simulink model "SF045A_HwAgSysArbn"  (R2013b)
settings: Solver=FixedStepDiscrete  SolverMode=SingleTasking  StartTime=0.0  StopTime=1  FixedStep=.002  RelTol=1e-3
values from neighbouring files (symbols this model uses):
  ARCHGLBPRM_2MILLISEC_SEC_F32 = DataDict.Constant    [SF045A_HwAgSysArbn_DataDict.m]
  ARCHGLBPRM_FLOATZEROTHD_ULS_F32 = DataDict.Constant    [SF045A_HwAgSysArbn_DataDict.m]
  ARCHGLBPRM_PIOVER180_ULS_F32 = DataDict.Constant    [SF045A_HwAgSysArbn_DataDict.m]
  CNVSECTOCNT_ULS_U32 = DataDict.Constant    [SF045A_HwAgSysArbn_DataDict.m]
  CNVTOMILLISEC_MILLISECPERCNT_F32 = DataDict.Constant    [SF045A_HwAgSysArbn_DataDict.m]
  FltInj_f32 = DataDict.Client    [SF045A_HwAgSysArbn_DataDict.m]
  FLTINJ_HWAGSYSARBN_HWAG = DataDict.Constant    [SF045A_HwAgSysArbn_DataDict.m]
  FLTINJ_HWAGSYSARBN_SERLCOMHWAG = DataDict.Constant    [SF045A_HwAgSysArbn_DataDict.m]
  HwAgCorrlnFlt = DataDict.NTC    [SF045A_HwAgSysArbn_DataDict.m]
  HwAgSnsrlsThdExcdd = DataDict.NTC    [SF045A_HwAgSysArbn_DataDict.m]
  HwAgSysArbnHwAgConf1Snsr = DataDict.Calibration    [SF045A_HwAgSysArbn_DataDict.m]
  HwAgSysArbnHwAgConf2Snsr = DataDict.Calibration    [SF045A_HwAgSysArbn_DataDict.m]
  HwAgSysArbnHwAgConfNoSnsr = DataDict.Calibration    [SF045A_HwAgSysArbn_DataDict.m]
  HwAgSysArbnHwAgCorrdCorrlnThd = DataDict.Calibration    [SF045A_HwAgSysArbn_DataDict.m]
  HwAgSysArbnHwAgCorrlnFailDebStep = DataDict.Calibration    [SF045A_HwAgSysArbn_DataDict.m]
  HwAgSysArbnHwAgCorrlnPassDebStep = DataDict.Calibration    [SF045A_HwAgSysArbn_DataDict.m]
  HwAgSysArbnHwAgCorrlnRng = DataDict.Calibration    [SF045A_HwAgSysArbn_DataDict.m]
  HwAgSysArbnHwAgSlewRate = DataDict.Calibration    [SF045A_HwAgSysArbn_DataDict.m]
  HwAgSysArbnHwAgSnsrlsCorrlnThd = DataDict.Calibration    [SF045A_HwAgSysArbn_DataDict.m]
  HwAgSysArbnHwAgSnsrlsKineThd = DataDict.Calibration    [SF045A_HwAgSysArbn_DataDict.m]
  HwAgSysArbnHwAgToMotAgCorrlnElpdTiLim = DataDict.Calibration    [SF045A_HwAgSysArbn_DataDict.m]
  HwAgSysArbnSerlComHwAgCorrdConf = DataDict.Calibration    [SF045A_HwAgSysArbn_DataDict.m]
  HwAgSysArbnSerlComHwAgSnsrlsConf = DataDict.Calibration    [SF045A_HwAgSysArbn_DataDict.m]
  HwAgSysArbnSlewRateTmr = DataDict.Calibration    [SF045A_HwAgSysArbn_DataDict.m]
  HWAGTHD_ULS_FLOAT32 = DataDict.Constant    [SF045A_HwAgSysArbn_DataDict.m]
  INVLDSRC_CNT_S08 = DataDict.Constant    [SF045A_HwAgSysArbn_DataDict.m]
  LRGSLEW_HWDEGPERSEC_F32 = DataDict.Constant    [SF045A_HwAgSysArbn_DataDict.m]
  NODEBSTEP_CNT_U16 = DataDict.Constant    [SF045A_HwAgSysArbn_DataDict.m]
  SLEWINPROGS_CNT_LGC = DataDict.Constant    [SF045A_HwAgSysArbn_DataDict.m]
  SLEWNOTINPROGS_CNT_LGC = DataDict.Constant    [SF045A_HwAgSysArbn_DataDict.m]
  SNSRDATASRCSELD_CNT_S08 = DataDict.Constant    [SF045A_HwAgSysArbn_DataDict.m]
  SNSRLSDATASRCSELD_CNT_S08 = DataDict.Constant    [SF045A_HwAgSysArbn_DataDict.m]
  SysGlbPrmSysKineRat = DataDict.ImprtdCal    [SF045A_HwAgSysArbn_DataDict.m]
  SysGlbPrmTorsBarStfn = DataDict.ImprtdCal    [SF045A_HwAgSysArbn_DataDict.m]
  ZEROTMR_MILLISEC_F32 = DataDict.Constant    [SF045A_HwAgSysArbn_DataDict.m]
undefined symbols (not defined in the file or in its folder): NtcSts1
libraries: NxtrLim x11, simulink x6, NxtrAbslt x6, Fil x3, autosarlib x2
(part 1 of 6)
settings Model: PauseTimes=0.48  CovFilter=UTP_SF045A_HwAgSysArbn_cov_flt_list  CovHTMLOptions=-sRT=1 -aTS=1 -bRG=1 -bTC=1 -hTR=0 -nFC=0 -scm=1 -bcm=1 -xEv=0  Creator=TZ5743  LastModifiedBy=NZ2883
settings SolverCC: AutoInsertRateTranBlk=on  InsertRTBMode=Always
settings DataIOCC: LimitDataPoints=off  SaveFormat=Structure  ReturnWorkspaceOutputs=on
settings OptimizationCC: BlockReduction=off  InlineParams=on  ZeroExternalMemoryAtStartup=off  ZeroInternalMemoryAtStartup=off  OptimizeModelRefInitCode=on  LifeSpan=1
settings DebuggingCC: SignalInfNanChecking=error  SignalRangeChecking=warning  UnderspecifiedInitializationDetection=Simplified  SolverPrmCheckMsg=error  InheritedTsInSrcMsg=error  DiscreteInheritContinuousMsg=error  SingleTaskRateTransMsg=error  TasksWithSamePriorityMsg=error  SigSpecEnsureSampleTimeMsg=error  CheckMatrixSingularityMsg=error  ParameterUnderflowMsg=error  ParameterPrecisionLossMsg=error  ParameterTunabilityLossMsg=error  FixptConstUnderflowMsg=warning  FixptConstOverflowMsg=warning  VectorMatrixConversionMsg=error  SignalLabelMismatchMsg=error  UnconnectedInputMsg=error  UnconnectedOutputMsg=error  UnconnectedLineMsg=error  SFcnCompatibilityMsg=error  UniqueDataStoreMsg=warning  BusObjectLabelMismatch=error  RootOutportRequireBusObject=error  AssertControl=DisableAll  ModelReferenceIOMsg=error  ModelReferenceVersionMismatchMessage=warning  ModelReferenceIOMismatchMessage=error  ModelReferenceCSMismatchMessage=warning  ModelReferenceDataLoggingMessage=error  StateNameClashWarn=warning  StrictBusMsg=ErrorOnBusTreatedAsVector  NonBusSignalsTreatedAsBus=error  SFUnexpectedBacktrackingDiag=error  SFInvalidInputDataAccessInChartInitDiag=error  SFNoUnconditionalDefaultTransitionDiag=error  SFTransitionOutsideNaturalParentDiag=error  SFUnconditionalTransitionShadowingDiag=error  SFUndirectedBroadcastEventsDiag=error
settings ModelReferenceCC: ModelReferenceNumInstancesAllowed=Single
settings RTWCC: SystemTargetFile=autosar.tlc  GenCodeOnly=on  TemplateMakefile=ert_default_tmf  Description=AUTOSAR  GenerateReport=on  ProcessScript=autosar_make_rtw_hook  LaunchReport=on
settings CodeAppCC: GenerateComments=off  IgnoreCustomStorageClasses=off  CustomSymbolStrType=$N$R$M  CustomSymbolStrBlkIO=$N$M  SimulinkBlockComments=off
settings STFCustomTargetCC: ParMdlRefBuildCompliant=on  CompOptLevelCompliant=on  IncludeMdlTerminateFcn=off  CombineOutputUpdateFcns=on  SuppressErrorStatus=on  ERTFirstTimeCompliant=on  ERTCustomFileBanners=on  SupportNonFinite=off  SupportComplex=off  SupportContinuousTime=off  SupportNonInlinedSFcns=off  MATLABClassNameForMDSCustomization=Simulink.SoftwareTarget.ERTCustomization  AutosarCompliant=on  GRTInterface=off  SystemTargetFile=autosar.tlc
settings ERTTargetCC: CodeReplacementLibrary=ANSI_C  ConcurrentExecutionCompliant=off  IncludeMdlTerminateFcn=off  SuppressErrorStatus=on  SupportNonFinite=off  SupportComplex=off  ModelStepFunctionPrototypeControlCompliant=off  CPPClassGenCompliant=off  AutosarCompliant=on  InlinedParameterPlacement=NonHierarchical  ERTCustomFileTemplate=example_file_process.tlc  EnableUserReplacementTypes=on

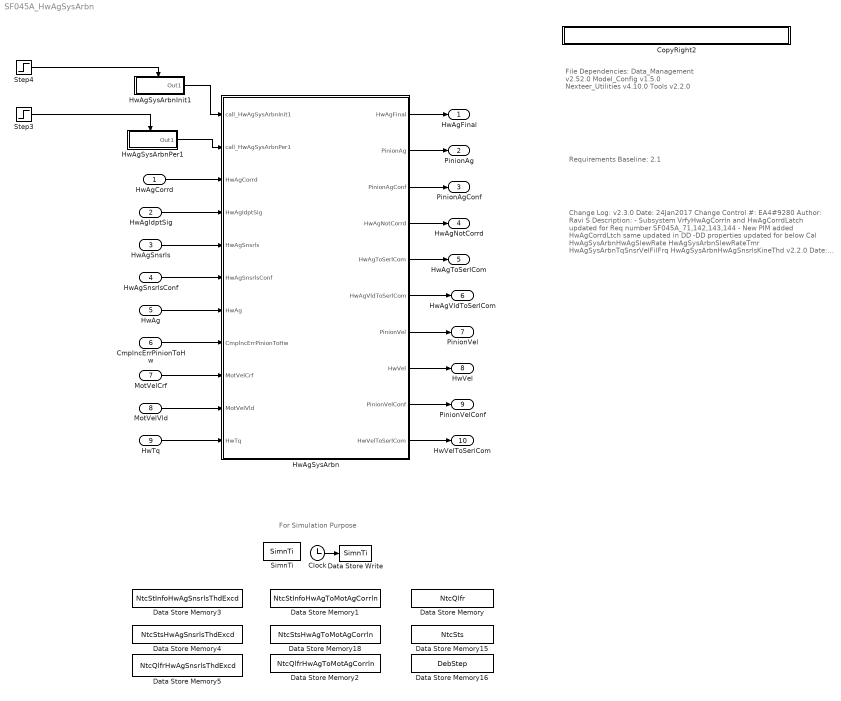
== system SF045A_HwAgSysArbn ==
  note: For Simulation Purpose
  note: File Dependencies:
      |
      | Data_Management v2.52.0
      | Model_Config v1.5.0
      | Nexteer_Utilities v4.10.0
      | Tools v2.2.0
  note: Requirements Baseline: 2.1
  note: Change Log:
      |
      | v2.3.0
      | Date: 24Jan2017
      | Change Control #: EA4#9280
      | Author: Ravi S
      | Description:
      | - Subsystem VrfyHwAgCorrln and HwAgCorrdLatch updated for
      |   Req number SF045A_71,142,143,144
      | - New PIM added HwAgCorrdLtch same updated in DD
      | -DD properties updated for below Cal
      |     HwAgSysArbnHwAgSlewRate
      |     HwAgSysArbnSlewRateTmr
      |     HwAgSysArbnTqSnsrVelFilFrq
      |     HwAgSysArbnHwAgSnsrlsKineThd
      |
      |
      | v2.2.0
      | Date: 29Nov2016
      | Change Control #: EA4#8582
      | Author: Ravi S
      | Description:
      | - MotorVelocityVld subsystem updated to compute
      |   HwVel = MotVelCrf / kinematic ratio.
      |
      |
      |
      |
      | v2.1.0
      | Date: 22-Nov-16
      | Change Control#: EA4#8179
      | Author:Ravi S
      | Description :
      | - Subsystem HwAgVelSeriCom and CalcPinionVel added .
      | - Subsystem HwAgSeriCom earlier was present in HwAgSrcSeln,
      |   which now repositioned  and added logig for Handwheel Velocity
      |   Serial Com.
      | - Requirements links added to all sub-systems
      |
      |
      | v2.0.0
      | Date: 15-Jun-16
      | Change Control#: EA4#5839
      | Author: Sudeep Shankar
      | Description :
      | - Generic design is now simplified considering only Pinion
      | coordinates to arbitrate the HwAg signals instead of flexibility to
      | choose between Handwheel, Pinion or MotorAg coordinates.
      | This resulted in removing the cals used to apply compilance error
      | compensation and priority selection.
      | - Kinematic Integrity diagonstic added
      | - HwAg to MotAg Correlation diagonstic added
      | - Logic added to arbitrate HwAg signal going to EOT when HwAg
      | sensor signals not available.
      |
      | v1.1.0
      | Date: 12-Sep-2015
      | Change Control #: EA4#860
      | Author:  Sudeep Shankar
      | Description:
      | - Minor modification in source change logic
      |  detection to avoid ambiguity in state variable
      |  read and write priorities
      | - Setting Initial condition of while loop to 'true'
      | instead of comparing greater than 1.
      | - Removed signal conversion blocks wherever
      | not required.
      | - Set while loop iteration to '-1' instead of restricting
      | it to '5' as condition check is in place to restrict
      | while iteration equal to number of signals present.
      |
      | v1.0.0
      | Date: 28-Aug-2015
      | Change Control #: EA4#860
      | Author:  Sudeep Shankar
      | Description:
      | - EA4 Initial Release
  HwAgCorrd : Inport  RequirementInfo={} %GIDa_cc9a7bcf_75f9_45c8_a24f_b8479fae80cf
  HwAgIdptSig : Inport  RequirementInfo={} %GIDa_9a7b919a_3c4b_44c1_bb96_545a47b8b3d3  Port=2
  HwAgSnsrls : Inport  RequirementInfo={} %GIDa_eede448f_64dd_4146_b16f_6fc16ca31f60  Port=3
  HwAgSnsrlsConf : Inport  RequirementInfo={} %GIDa_f6d9b3ed_9576_46cf_8319_2d07116884b2  Port=4
  HwAg : Inport  RequirementInfo={} %GIDa_3ab8439e_d791_45cf_9b38_dc1d6a5d96c4  Port=5
  CmplncErrPinionToHw : Inport  RequirementInfo={} %GIDa_8afc3a2b_29a0_4b25_ac8f_049b17fb3d6a  Port=6
  MotVelCrf : Inport  Port=7
  MotVelVld : Inport  Port=8
  HwTq : Inport  Port=9
  Clock : Clock
  CopyRight2 : Subsystem  Description=|  mask(Copyright Information){none=on}
      | Copyright info block.                                               
      |                                                                     
      | Place copyright information at the top of every subsystem in design.
      mask prompts: none "No parameters"
      mask help: Place copyright information at the top of every subsystem in design.
      mask Display:
      | NxtrConf = 'Nexteer Confidential';
      | 
      | sys = bdroot; %handle for the current model ("system")
      | first = get_param(sys,'Created');
      | first = first(end-3:end);  %year is last four digits
      | 
      | last = get_param(sys,'LastModifiedDate');
      | if isempty(last)
      |     last = datestr(now,'yyyy');
      | else
      |     last = last(end-3:end);
      | end
      | 
      | if strcmp(first,last)
      |     fprintf('%s -- Copyright %s Nexteer',NxtrConf,first)
      | else
      |     fprintf('%s -- %s%s- %s Nexteer',NxtrConf,char(169),first,last)
      | end
  Data Store Memory : DataStoreMemory  DataStoreName=NtcQlfr  InitialValue=SigQlfr1.SIGQLFR_NORES  OutDataTypeStr=Enum: SigQlfr1
  Data Store Memory1 : DataStoreMemory  DataStoreName=NtcStInfoHwAgToMotAgCorrln  OutDataTypeStr=uint8
  Data Store Memory15 : DataStoreMemory  DataStoreName=NtcSts  InitialValue=NtcSts1.NTCSTS_PREPASSD  OutDataTypeStr=Enum: NtcSts1
  Data Store Memory16 : DataStoreMemory  DataStoreName=DebStep
  Data Store Memory18 : DataStoreMemory  DataStoreName=NtcStsHwAgToMotAgCorrln  InitialValue=NtcSts1.NTCSTS_PASSD  OutDataTypeStr=Enum: NtcSts1
  Data Store Memory2 : DataStoreMemory  DataStoreName=NtcQlfrHwAgToMotAgCorrln  InitialValue=SigQlfr1.SIGQLFR_NORES  OutDataTypeStr=Enum: SigQlfr1
  Data Store Memory3 : DataStoreMemory  DataStoreName=NtcStInfoHwAgSnsrlsThdExcd  OutDataTypeStr=uint8
  Data Store Memory4 : DataStoreMemory  DataStoreName=NtcStsHwAgSnsrlsThdExcd  InitialValue=NtcSts1.NTCSTS_PASSD  OutDataTypeStr=Enum: NtcSts1
  Data Store Memory5 : DataStoreMemory  DataStoreName=NtcQlfrHwAgSnsrlsThdExcd  InitialValue=SigQlfr1.SIGQLFR_NORES  OutDataTypeStr=Enum: SigQlfr1
  Data Store Write : DataStoreWrite  DataStoreName=SimnTi
  HwAgSysArbn : Subsystem  RequirementInfo="{'linktype_rmi_doors' '00012ce0 (/E-STEER Core/SubSystem Specifications/Application Functions - EA4/SF045A Handwheel Angle System Arbitration)' '#SF045A_108' 'true' 'REQ:  SF045A_108' '' } %GIDa_b3e0ed6f_fb94_4fa4_96b1_04061689a89e"
  HwAgSysArbnInit1 : Subsystem  RequirementInfo="{'linktype_rmi_doors' '00012ce0 (/E-STEER Core/SubSystem Specifications/Application Functions - EA4/SF045A Handwheel Angle System Arbitration)' '#SF045A_108' 'true' 'REQ:  SF045A_108' '' ; 'linktype_rmi_doors' '00012ce0 (/E-STEER Core/SubSystem Specifications/Application Functions - EA4/SF045A Handwheel Angle System Arbitration)' '#SF045A_34' 'true' 'REQ:  SF045A_34' '' } %GIDa_057ddbd1_6821_4128_a5e6_a444f48d7204"  TreatAsAtomicUnit=on
  HwAgSysArbnPer1 : Subsystem  RequirementInfo="{'linktype_rmi_doors' '00012ce0 (/E-STEER Core/SubSystem Specifications/Application Functions - EA4/SF045A Handwheel Angle System Arbitration)' '#SF045A_108' 'true' 'REQ:  SF045A_108' '' ; 'linktype_rmi_doors' '00012ce0 (/E-STEER Core/SubSystem Specifications/Application Functions - EA4/SF045A Handwheel Angle System Arbitration)' '#SF045A_34' 'true' 'REQ:  SF045A_34' '' } %GIDa_e117302a_b889_4d12_a49a_80c3f747018f"  TreatAsAtomicUnit=on
  SimnTi : DataStoreMemory  DataStoreName=SimnTi
  Step3 : Step  Time=0  SampleTime=0.002
  Step4 : Step  Time=0  Before=1  After=0  SampleTime=0.002
  HwAgFinal : Outport
  PinionAg : Outport  Port=2
  PinionAgConf : Outport  Port=3
  HwAgNotCorrd : Outport  Port=4
  HwAgToSerlCom : Outport  Port=5
  HwAgVldToSerlCom : Outport  Port=6
  PinionVel : Outport  Port=7
  HwVel : Outport  Port=8
  PinionVelConf : Outport  Port=9
  HwVelToSeriCom : Outport  Port=10
  wires:
  HwAgSysArbn/2(PinionAg) -> PinionAg/1
  HwAgSysArbn/3(PinionAgConf) -> PinionAgConf/1
  HwAgSysArbn/4(HwAgNotCorrd) -> HwAgNotCorrd/1
  HwAgSysArbn/1(HwAgFinal) -> HwAgFinal/1
  HwAgSysArbn/6(HwAgVldToSerlCom) -> HwAgVldToSerlCom/1
  Clock/1 -> Data Store Write/1
  HwAgSysArbn/5(HwAgToSerlCom) -> HwAgToSerlCom/1
  HwAgSysArbnInit1/1(Out1) -> HwAgSysArbn/1(call_HwAgSysArbnInit1)
  HwAgSysArbnPer1/1(Out1) -> HwAgSysArbn/2(call_HwAgSysArbnPer1)
  HwAgSnsrls/1 -> HwAgSysArbn/5(HwAgSnsrls)
  HwAgCorrd/1 -> HwAgSysArbn/3(HwAgCorrd)
  HwAgSnsrlsConf/1 -> HwAgSysArbn/6(HwAgSnsrlsConf)
  HwAgIdptSig/1 -> HwAgSysArbn/4(HwAgIdptSig)
  CmplncErrPinionToHw/1 -> HwAgSysArbn/8(CmplncErrPinionToHw)
  HwAg/1 -> HwAgSysArbn/7(HwAg)
  Step3/1 -> HwAgSysArbnPer1/Enable
  MotVelCrf/1 -> HwAgSysArbn/9(MotVelCrf)
  MotVelVld/1 -> HwAgSysArbn/10(MotVelVld)
  HwTq/1 -> HwAgSysArbn/11(HwTq)
  HwAgSysArbn/7(PinionVel) -> PinionVel/1
  HwAgSysArbn/8(HwVel) -> HwVel/1
  HwAgSysArbn/9(PinionVelConf) -> PinionVelConf/1
  HwAgSysArbn/10(HwVelToSerlCom) -> HwVelToSeriCom/1
  Step4/1 -> HwAgSysArbnInit1/Enable

== system SF045A_HwAgSysArbn/CopyRight2 ==

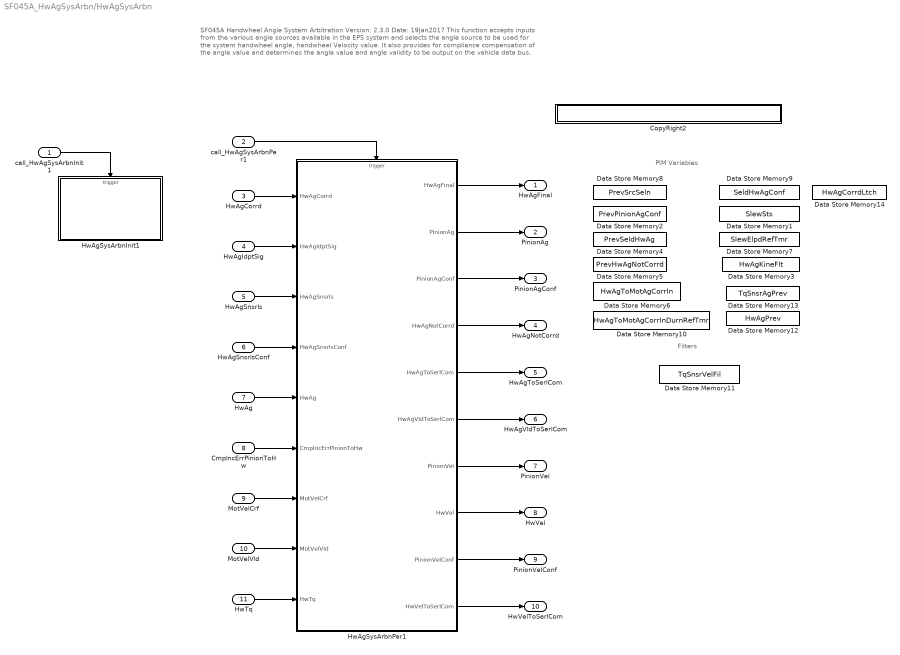
== system SF045A_HwAgSysArbn/HwAgSysArbn ==
  note: PIM Variables
  note: SF045A  Handwheel Angle System Arbitration       Version: 2.3.0                                                        Date: 19Jan2017
      |
      | This function accepts inputs from the various angle sources available in the EPS system and selects the angle
      | source to be used for the system handwheel angle, handwheel Velocity value.
      | It also provides for compliance compensation of the angle value and determines the angle value and angle validity to be output on the vehicle data bus.
  note: Filters
  call_HwAgSysArbnInit1 : Inport
  call_HwAgSysArbnPer1 : Inport  Port=2
  HwAgCorrd : Inport  RequirementInfo="{'linktype_rmi_doors' '00012ce0 (/E-STEER Core/SubSystem Specifications/Application Functions - EA4/SF045A Handwheel Angle System Arbitration)' '#SF045A_9' 'true' 'REQ:  SF045A_9' '' } %GIDa_0c48395d_f55e_4aa8_967c_ddfcd5dc0f09"  Port=3
  HwAgIdptSig : Inport  RequirementInfo="{'linktype_rmi_doors' '00012ce0 (/E-STEER Core/SubSystem Specifications/Application Functions - EA4/SF045A Handwheel Angle System Arbitration)' '#SF045A_47' 'true' 'REQ:  SF045A_47' '' } %GIDa_050c3700_87b8_4e6a_a603_fe10bf5bb98d"  Port=4
  HwAgSnsrls : Inport  RequirementInfo="{'linktype_rmi_doors' '00012ce0 (/E-STEER Core/SubSystem Specifications/Application Functions - EA4/SF045A Handwheel Angle System Arbitration)' '#SF045A_46' 'true' 'REQ:  SF045A_46' '' } %GIDa_2af70a6d_5cf9_42e5_985f_0de67760f974"  Port=5
  HwAgSnsrlsConf : Inport  RequirementInfo="{'linktype_rmi_doors' '00012ce0 (/E-STEER Core/SubSystem Specifications/Application Functions - EA4/SF045A Handwheel Angle System Arbitration)' '#SF045A_48' 'true' 'REQ:  SF045A_48' '' } %GIDa_205f4441_a425_4e75_91eb_166c28519f31"  Port=6
  HwAg : Inport  RequirementInfo="{'linktype_rmi_doors' '00012ce0 (/E-STEER Core/SubSystem Specifications/Application Functions - EA4/SF045A Handwheel Angle System Arbitration)' '#SF045A_49' 'true' 'REQ:  SF045A_49' '' } %GIDa_bd860903_e40a_4856_a107_6e65debfd627"  Port=7
  CmplncErrPinionToHw : Inport  RequirementInfo="{'linktype_rmi_doors' '00012ce0 (/E-STEER Core/SubSystem Specifications/Application Functions - EA4/SF045A Handwheel Angle System Arbitration)' '#SF045A_50' 'true' 'REQ:  SF045A_50' '' } %GIDa_fd50d5ef_7c8c_43a4_8956_a275e6267051"  Port=8
  MotVelCrf : Inport  RequirementInfo="{'linktype_rmi_doors' '00012ce0 (/E-STEER Core/SubSystem Specifications/Application Functions - EA4/SF045A Handwheel Angle System Arbitration)' '#SF045A_127' 'true' 'REQ:  SF045A_127' '' } %GIDa_90030ca0_2589_4eab_adf5_a0272c142c23"  Port=9
  MotVelVld : Inport  RequirementInfo="{'linktype_rmi_doors' '00012ce0 (/E-STEER Core/SubSystem Specifications/Application Functions - EA4/SF045A Handwheel Angle System Arbitration)' '#SF045A_128' 'true' 'REQ:  SF045A_128' '' } %GIDa_c2b99d6a_26e3_4ced_a354_7c878afdb5f5"  Port=10
  HwTq : Inport  RequirementInfo="{'linktype_rmi_doors' '00012ce0 (/E-STEER Core/SubSystem Specifications/Application Functions - EA4/SF045A Handwheel Angle System Arbitration)' '#SF045A_130' 'true' 'REQ:  SF045A_130' '' } %GIDa_722f0d6d_b063_4bab_a5a3_bad3ad3ad2ff"  Port=11
  CopyRight2 : Subsystem  Description=|  mask(Copyright Information){none=on}
      | Copyright info block.                                               
      |                                                                     
      | Place copyright information at the top of every subsystem in design.
      mask prompts: none "No parameters"
      mask help: Place copyright information at the top of every subsystem in design.
      mask Display:
      | NxtrConf = 'Nexteer Confidential';
      | 
      | sys = bdroot; %handle for the current model ("system")
      | first = get_param(sys,'Created');
      | first = first(end-3:end);  %year is last four digits
      | 
      | last = get_param(sys,'LastModifiedDate');
      | if isempty(last)
      |     last = datestr(now,'yyyy');
      | else
      |     last = last(end-3:end);
      | end
      | 
      | if strcmp(first,last)
      |     fprintf('%s -- Copyright %s Nexteer',NxtrConf,first)
      | else
      |     fprintf('%s -- %s%s- %s Nexteer',NxtrConf,char(169),first,last)
      | end
  Data Store Memory1 : DataStoreMemory  DataStoreName=SlewSts  StateMustResolveToSignalObject=on
  Data Store Memory10 : DataStoreMemory  DataStoreName=HwAgToMotAgCorrlnDurnRefTmr  StateMustResolveToSignalObject=on
  Data Store Memory11 : DataStoreMemory  DataStoreName=TqSnsrVelFil  InitialValue=[]  OutDataTypeStr=Bus: FilLpRec1  StateMustResolveToSignalObject=on
  Data Store Memory12 : DataStoreMemory  DataStoreName=HwAgPrev  StateMustResolveToSignalObject=on
  Data Store Memory13 : DataStoreMemory  DataStoreName=TqSnsrAgPrev  StateMustResolveToSignalObject=on
  Data Store Memory14 : DataStoreMemory  DataStoreName=HwAgCorrdLtch  StateMustResolveToSignalObject=on
  Data Store Memory2 : DataStoreMemory  DataStoreName=PrevPinionAgConf  StateMustResolveToSignalObject=on
  Data Store Memory3 : DataStoreMemory  DataStoreName=HwAgKineFlt  StateMustResolveToSignalObject=on
  Data Store Memory4 : DataStoreMemory  DataStoreName=PrevSeldHwAg  StateMustResolveToSignalObject=on
  Data Store Memory5 : DataStoreMemory  DataStoreName=PrevHwAgNotCorrd  StateMustResolveToSignalObject=on
  Data Store Memory6 : DataStoreMemory  DataStoreName=HwAgToMotAgCorrln  StateMustResolveToSignalObject=on
  Data Store Memory7 : DataStoreMemory  DataStoreName=SlewElpdRefTmr  StateMustResolveToSignalObject=on
  Data Store Memory8 : DataStoreMemory  DataStoreName=PrevSrcSeln  StateMustResolveToSignalObject=on
  Data Store Memory9 : DataStoreMemory  DataStoreName=SeldHwAgConf  StateMustResolveToSignalObject=on
  HwAgSysArbnInit1 : Subsystem  RequirementInfo="{'linktype_rmi_doors' '00012ce0 (/E-STEER Core/SubSystem Specifications/Application Functions - EA4/SF045A Handwheel Angle System Arbitration)' '#SF045A_34' 'true' 'REQ:  SF045A_34' '' ; 'linktype_rmi_doors' '00012ce0 (/E-STEER Core/SubSystem Specifications/Application Functions - EA4/SF045A Handwheel Angle System Arbitration)' '#SF045A_123' 'true' 'REQ:  SF045A_123' '' } %GIDa_ffe1340e_7dd3_453f_8ec7_9bdff50c1f90"  TreatAsAtomicUnit=on
  HwAgSysArbnPer1 : Subsystem  RequirementInfo="{'linktype_rmi_doors' '00012ce0 (/E-STEER Core/SubSystem Specifications/Application Functions - EA4/SF045A Handwheel Angle System Arbitration)' '#SF045A_67' 'true' 'REQ:  SF045A_67' '' } %GIDa_40c16d0c_868c_4be8_ac7a_d7644aab2a82"
  HwAgFinal : Outport  RequirementInfo="{'linktype_rmi_doors' '00012ce0 (/E-STEER Core/SubSystem Specifications/Application Functions - EA4/SF045A Handwheel Angle System Arbitration)' '#SF045A_11' 'true' 'REQ:  SF045A_11' '' } %GIDa_011fe0ec_bcc0_4a9e_bfa8_b93370ffdc5f"
  PinionAg : Outport  RequirementInfo="{'linktype_rmi_doors' '00012ce0 (/E-STEER Core/SubSystem Specifications/Application Functions - EA4/SF045A Handwheel Angle System Arbitration)' '#SF045A_51' 'true' 'REQ:  SF045A_51' '' } %GIDa_f176d339_cae7_40f0_af7d_2598900e3a6e"  Port=2
  PinionAgConf : Outport  RequirementInfo="{'linktype_rmi_doors' '00012ce0 (/E-STEER Core/SubSystem Specifications/Application Functions - EA4/SF045A Handwheel Angle System Arbitration)' '#SF045A_52' 'true' 'REQ:  SF045A_52' '' } %GIDa_ba6f2b72_e674_40ee_820e_69cfc9bdaacd"  Port=3
  HwAgNotCorrd : Outport  RequirementInfo="{'linktype_rmi_doors' '00012ce0 (/E-STEER Core/SubSystem Specifications/Application Functions - EA4/SF045A Handwheel Angle System Arbitration)' '#SF045A_55' 'true' 'REQ:  SF045A_55' '' } %GIDa_667dfd31_56c6_4848_b6a8_5a3d7a5632fb"  Port=4
  HwAgToSerlCom : Outport  RequirementInfo="{'linktype_rmi_doors' '00012ce0 (/E-STEER Core/SubSystem Specifications/Application Functions - EA4/SF045A Handwheel Angle System Arbitration)' '#SF045A_56' 'true' 'REQ:  SF045A_56' '' } %GIDa_8096249c_a6e2_4a31_b51a_c06af36d6bde"  Port=5
  HwAgVldToSerlCom : Outport  RequirementInfo="{'linktype_rmi_doors' '00012ce0 (/E-STEER Core/SubSystem Specifications/Application Functions - EA4/SF045A Handwheel Angle System Arbitration)' '#SF045A_57' 'true' 'REQ:  SF045A_57' '' } %GIDa_30b9e9dd_ad37_434a_8538_15d621b4541c"  Port=6
  PinionVel : Outport  RequirementInfo="{'linktype_rmi_doors' '00012ce0 (/E-STEER Core/SubSystem Specifications/Application Functions - EA4/SF045A Handwheel Angle System Arbitration)' '#SF045A_132' 'true' 'REQ:  SF045A_132' '' } %GIDa_825df61a_9b42_4745_9a19_f867d9578a4d"  Port=7
  HwVel : Outport  RequirementInfo="{'linktype_rmi_doors' '00012ce0 (/E-STEER Core/SubSystem Specifications/Application Functions - EA4/SF045A Handwheel Angle System Arbitration)' '#SF045A_134' 'true' 'REQ:  SF045A_134' '' } %GIDa_df719774_fce7_4f7c_868b_fd6ca13ffd9c"  Port=8
  PinionVelConf : Outport  RequirementInfo="{'linktype_rmi_doors' '00012ce0 (/E-STEER Core/SubSystem Specifications/Application Functions - EA4/SF045A Handwheel Angle System Arbitration)' '#SF045A_133' 'true' 'REQ:  SF045A_133' '' } %GIDa_5297214b_1fb7_41a8_8266_2143d92809ac"  Port=9
  HwVelToSerlCom : Outport  RequirementInfo="{'linktype_rmi_doors' '00012ce0 (/E-STEER Core/SubSystem Specifications/Application Functions - EA4/SF045A Handwheel Angle System Arbitration)' '#SF045A_135' 'true' 'REQ:  SF045A_135' '' } %GIDa_0c50da69_21aa_4d0e_a4ce_f9ea2be8a725"  Port=10
  wires:
  call_HwAgSysArbnPer1/1 -> HwAgSysArbnPer1/Trigger
  call_HwAgSysArbnInit1/1 -> HwAgSysArbnInit1/Trigger
  HwAgSysArbnPer1/4(HwAgNotCorrd) -> HwAgNotCorrd/1
  HwAgSysArbnPer1/2(PinionAg) -> PinionAg/1
  HwAgSysArbnPer1/6(HwAgVldToSerlCom) -> HwAgVldToSerlCom/1
  HwAgSysArbnPer1/5(HwAgToSerlCom) -> HwAgToSerlCom/1
  HwAgSysArbnPer1/3(PinionAgConf) -> PinionAgConf/1
  HwAgSnsrls/1 -> HwAgSysArbnPer1/3(HwAgSnsrls)
  HwAgCorrd/1 -> HwAgSysArbnPer1/1(HwAgCorrd)
  HwAgSnsrlsConf/1 -> HwAgSysArbnPer1/4(HwAgSnsrlsConf)
  HwAgIdptSig/1 -> HwAgSysArbnPer1/2(HwAgIdptSig)
  CmplncErrPinionToHw/1 -> HwAgSysArbnPer1/6(CmplncErrPinionToHw)
  HwAg/1 -> HwAgSysArbnPer1/5(HwAg)
  HwAgSysArbnPer1/1(HwAgFinal) -> HwAgFinal/1
  MotVelCrf/1 -> HwAgSysArbnPer1/7(MotVelCrf)
  MotVelVld/1 -> HwAgSysArbnPer1/8(MotVelVld)
  HwTq/1 -> HwAgSysArbnPer1/9(HwTq)
  HwAgSysArbnPer1/7(PinionVel) -> PinionVel/1
  HwAgSysArbnPer1/8(HwVel) -> HwVel/1
  HwAgSysArbnPer1/9(PinionVelConf) -> PinionVelConf/1
  HwAgSysArbnPer1/10(HwVelToSerlCom) -> HwVelToSerlCom/1

== system SF045A_HwAgSysArbn/HwAgSysArbnInit1 ==
  Enable : EnablePort
  CopyRight2 : Subsystem  Description=|  mask(Copyright Information){none=on}
      | Copyright info block.                                               
      |                                                                     
      | Place copyright information at the top of every subsystem in design.
      mask prompts: none "No parameters"
      mask help: Place copyright information at the top of every subsystem in design.
      mask Display:
      | NxtrConf = 'Nexteer Confidential';
      | 
      | sys = bdroot; %handle for the current model ("system")
      | first = get_param(sys,'Created');
      | first = first(end-3:end);  %year is last four digits
      | 
      | last = get_param(sys,'LastModifiedDate');
      | if isempty(last)
      |     last = datestr(now,'yyyy');
      | else
      |     last = last(end-3:end);
      | end
      | 
      | if strcmp(first,last)
      |     fprintf('%s -- Copyright %s Nexteer',NxtrConf,first)
      | else
      |     fprintf('%s -- %s%s- %s Nexteer',NxtrConf,char(169),first,last)
      | end
  Function-Call Generator : simulink/Ports & Subsystems/Function-Call Generator  sample_time=0.002  numberOfIterations=1
  Out1 : Outport
  wires:
  Function-Call Generator/1 -> Out1/1

== system SF045A_HwAgSysArbn/HwAgSysArbnPer1 ==
  Enable : EnablePort
  CopyRight2 : Subsystem  Description=|  mask(Copyright Information){none=on}
      | Copyright info block.                                               
      |                                                                     
      | Place copyright information at the top of every subsystem in design.
      mask prompts: none "No parameters"
      mask help: Place copyright information at the top of every subsystem in design.
      mask Display:
      | NxtrConf = 'Nexteer Confidential';
      | 
      | sys = bdroot; %handle for the current model ("system")
      | first = get_param(sys,'Created');
      | first = first(end-3:end);  %year is last four digits
      | 
      | last = get_param(sys,'LastModifiedDate');
      | if isempty(last)
      |     last = datestr(now,'yyyy');
      | else
      |     last = last(end-3:end);
      | end
      | 
      | if strcmp(first,last)
      |     fprintf('%s -- Copyright %s Nexteer',NxtrConf,first)
      | else
      |     fprintf('%s -- %s%s- %s Nexteer',NxtrConf,char(169),first,last)
      | end
  call_HwAgSysArbnPer1 : simulink/Ports & Subsystems/Function-Call Generator  RequirementInfo={} %GIDa_ec825fb2_121b_4b6b_b290_bf31fce876d3  sample_time=0.002  numberOfIterations=1
  Out1 : Outport
  wires:
  call_HwAgSysArbnPer1/1 -> Out1/1

== system SF045A_HwAgSysArbn/HwAgSysArbn/CopyRight2 ==

== system SF045A_HwAgSysArbn/HwAgSysArbn/HwAgSysArbnInit1 ==
  note: Set Kinematic Integrity Diagostic to PASS
  note: 'PrevSrcSeln' is set to "INVALID SOURCE" in initialization to ensure that source change is detected
      | when source selection happens for the first time after initialization.
  note: Initialize Slew State to "Not in progress" at startup
  function : TriggerPort  TriggerType=function-call
  Constant1 : Constant  RequirementInfo={} %GIDa_bd6cf35a_c752_43ca_93be_9c9b276a6240  Value=0
  Constant2 : Constant  RequirementInfo={} %GIDa_50809f46_4379_44ea_9224_8e996deda18f  Value=NODEBSTEP_CNT_U16
  Constant3 : Constant  RequirementInfo={} %GIDa_566596cf_6e44_474c_b09e_09702d851a46  Value=HwAgSnsrlsThdExcdd
  Constant7 : Constant  Value=SLEWNOTINPROGS_CNT_LGC
  CopyRight2 : Subsystem  Description=|  mask(Copyright Information){none=on}
      | Copyright info block.                                               
      |                                                                     
      | Place copyright information at the top of every subsystem in design.
      mask prompts: none "No parameters"
      mask help: Place copyright information at the top of every subsystem in design.
      mask Display:
      | NxtrConf = 'Nexteer Confidential';
      | 
      | sys = bdroot; %handle for the current model ("system")
      | first = get_param(sys,'Created');
      | first = first(end-3:end);  %year is last four digits
      | 
      | last = get_param(sys,'LastModifiedDate');
      | if isempty(last)
      |     last = datestr(now,'yyyy');
      | else
      |     last = last(end-3:end);
      | end
      | 
      | if strcmp(first,last)
      |     fprintf('%s -- Copyright %s Nexteer',NxtrConf,first)
      | else
      |     fprintf('%s -- %s%s- %s Nexteer',NxtrConf,char(169),first,last)
      | end
  Data Store Write1 : DataStoreWrite  RequirementInfo={} %GIDa_ed78b567_a6b6_41da_bf60_9df352ceaf90  DataStoreName=HwAgToMotAgCorrlnDurnRefTmr
  Data Store Write5 : DataStoreWrite  RequirementInfo={} %GIDa_5976233f_3450_4a81_8e0a_eaaf4d56a88e  DataStoreName=SlewSts
  Data Store Write6 : DataStoreWrite  RequirementInfo={} %GIDa_4cb2551e_dfbf_4575_8209_178b050baa05  DataStoreName=PrevSrcSeln
  Enumerated Constant1 : simulink/Sources/Enumerated Constant  RequirementInfo={} %GIDa_78dbafe2_a67d_4f00_b984_ee6afb604272  OutDataTypeStr=Enum: NtcSts1  Value=NtcSts1.NTCSTS_PASSD  SampleTime=inf
  GetRefTmr100MicroSec32bit : Subsystem  RequirementInfo={} %GIDa_f5914e2f_3dac_4251_b655_ba1168612562
  Kinematic Integrity : Subsystem  RequirementInfo={} %GIDa_e2a8d71c_6639_4a30_b92d_fbf0b44b7e0b  mask(SetNTC){}
      mask help: SetNTC library block
  SET1 : Constant  RequirementInfo={} %GIDa_173d0037_1d29_4d18_8e95_d80bd9f8e211  Value=INVLDSRC_CNT_S08
  TqSnsrVelFil : Fil/FilLpInit  Ic=0  Ts=ARCHGLBPRM_2MILLISEC_SEC_F32  Freq=HwAgSysArbnTqSnsrVelFilFrq  StVar=TqSnsrVelFil
  wires:
  Constant7/1 -> Data Store Write5/1
  SET1/1 -> Data Store Write6/1
  Enumerated Constant1/1 -> Kinematic Integrity/3(NtcSts)
  Constant1/1 -> Kinematic Integrity/2(NtcStInfo)
  Constant3/1 -> Kinematic Integrity/1(NtcNr)
  Constant2/1 -> Kinematic Integrity/4(DebStep)
  GetRefTmr100MicroSec32bit/1(RefTmr) -> Data Store Write1/1

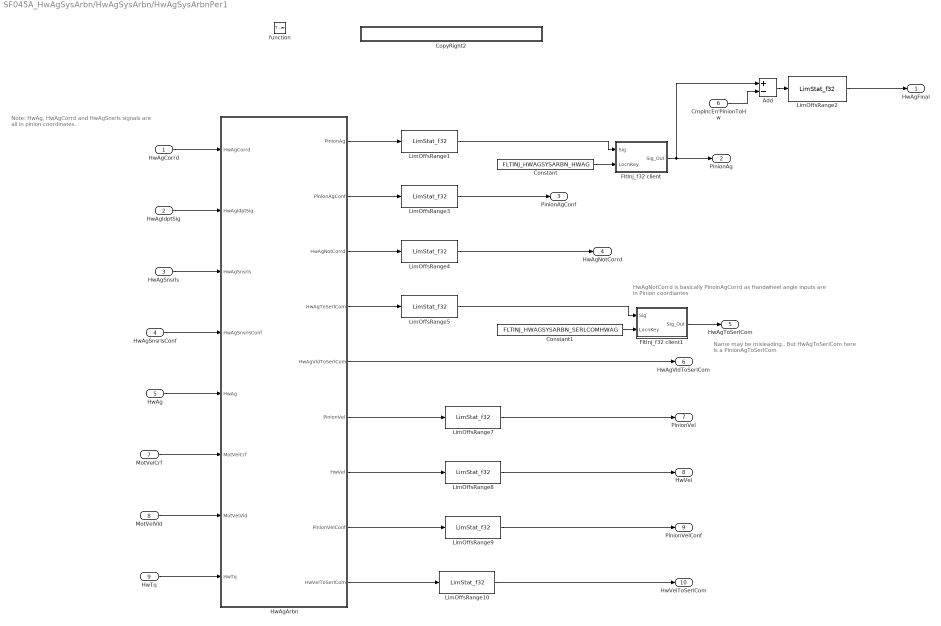
== system SF045A_HwAgSysArbn/HwAgSysArbn/HwAgSysArbnPer1 ==
  note: Name may be misleading..
      | But HwAgToSerlCom here is a PinionAgToSerlCom
  note: HwAgNotCorrd is basically PinoinAgCorrd as Handwheel angle inputs
      | are in Pinion coordiantes
  note: Note: HwAg, HwAgCorrd and HwAgSnsrls signals
      | are all in pinion coordinates.
  HwAgCorrd : Inport
  HwAgIdptSig : Inport  Port=2
  HwAgSnsrls : Inport  Port=3
  HwAgSnsrlsConf : Inport  Port=4
  HwAg : Inport  Port=5
  CmplncErrPinionToHw : Inport  Port=6
  MotVelCrf : Inport  Port=7
  MotVelVld : Inport  Port=8
  HwTq : Inport  Port=9
  function : TriggerPort  TriggerType=function-call
  Add : Sum  RequirementInfo="{'linktype_rmi_doors' '00012ce0 (/E-STEER Core/SubSystem Specifications/Application Functions - EA4/SF045A Handwheel Angle System Arbitration)' '#SF045A_112' 'true' 'REQ:  SF045A_112' '' } %GIDa_2d6cc4c3_3517_4898_866f_2c6dc4253050"  Inputs=+-
  Constant : Constant  RequirementInfo="{'linktype_rmi_doors' '00012ce0 (/E-STEER Core/SubSystem Specifications/Application Functions - EA4/SF045A Handwheel Angle System Arbitration)' '#SF045A_110' 'true' 'REQ:  SF045A_110' '' } %GIDa_a52d7649_e318_4faa_96ee_a31dcdf91c61"  Value=FLTINJ_HWAGSYSARBN_HWAG
  Constant1 : Constant  RequirementInfo="{'linktype_rmi_doors' '00012ce0 (/E-STEER Core/SubSystem Specifications/Application Functions - EA4/SF045A Handwheel Angle System Arbitration)' '#SF045A_110' 'true' 'REQ:  SF045A_110' '' } %GIDa_07ff8395_6a89_418d_9d3e_d1c6e454756f"  Value=FLTINJ_HWAGSYSARBN_SERLCOMHWAG
  CopyRight2 : Subsystem  Description=|  mask(Copyright Information){none=on}
      | Copyright info block.                                               
      |                                                                     
      | Place copyright information at the top of every subsystem in design.
      mask prompts: none "No parameters"
      mask help: Place copyright information at the top of every subsystem in design.
      mask Display:
      | NxtrConf = 'Nexteer Confidential';
      | 
      | sys = bdroot; %handle for the current model ("system")
      | first = get_param(sys,'Created');
      | first = first(end-3:end);  %year is last four digits
      | 
      | last = get_param(sys,'LastModifiedDate');
      | if isempty(last)
      |     last = datestr(now,'yyyy');
      | else
      |     last = last(end-3:end);
      | end
      | 
      | if strcmp(first,last)
      |     fprintf('%s -- Copyright %s Nexteer',NxtrConf,first)
      | else
      |     fprintf('%s -- %s%s- %s Nexteer',NxtrConf,char(169),first,last)
      | end
  FltInj_f32 client : Subsystem  RequirementInfo="{'linktype_rmi_doors' '00012ce0 (/E-STEER Core/SubSystem Specifications/Application Functions - EA4/SF045A Handwheel Angle System Arbitration)' '#SF045A_110' 'true' 'REQ:  SF045A_110' '' } %GIDa_9135daa6_faf3_4380_ac44_151a9c0b94f1"  Variant=on  OverrideUsingVariant=FLTINJENA ~= STD_ON
      settings: GeneratePreprocessorConditionals=on
  FltInj_f32 client1 : Subsystem  RequirementInfo="{'linktype_rmi_doors' '00012ce0 (/E-STEER Core/SubSystem Specifications/Application Functions - EA4/SF045A Handwheel Angle System Arbitration)' '#SF045A_111' 'true' 'REQ:  SF045A_111' '' } %GIDa_77ed299a_7809_433b_8d2d_dd385f0e6e22"  Variant=on  OverrideUsingVariant=FLTINJENA ~= STD_ON
      settings: GeneratePreprocessorConditionals=on
  HwAgArbn : Subsystem
  LimOffsRange1 : NxtrLim/LimStat_f32  LoLim=PINIONAGLOWLIM_HWDEG_F32  HiLim=PINIONAGHILIM_HWDEG_F32
      settings: AttributesFormatString=|
      | Low Limit: %<LoLim>
      | High Limit:%<HiLim>
  LimOffsRange10 : NxtrLim/LimStat_f32  LoLim=HWVELLOWLIM_HWRADPERSEC_F32  HiLim=HWVELHILIM_HWRADPERSEC_F32
      settings: AttributesFormatString=|
      | Low Limit: %<LoLim>
      | High Limit:%<HiLim>
  LimOffsRange2 : NxtrLim/LimStat_f32  RequirementInfo="{'linktype_rmi_doors' '00012ce0 (/E-STEER Core/SubSystem Specifications/Application Functions - EA4/SF045A Handwheel Angle System Arbitration)' '#SF045A_112' 'true' 'REQ:  SF045A_112' '' } %GIDa_b3dcb40f_224d_4843_a30f_9c254bb42720"  LoLim=PINIONAGLOWLIM_HWDEG_F32  HiLim=PINIONAGHILIM_HWDEG_F32
      settings: AttributesFormatString=|
      | Low Limit: %<LoLim>
      | High Limit:%<HiLim>
  LimOffsRange3 : NxtrLim/LimStat_f32  LoLim=PINIONAGCONFLOWLIM_ULS_F32  HiLim=PINIONAGCONFHILIM_ULS_F32
      settings: AttributesFormatString=|
      | Low Limit: %<LoLim>
      | High Limit:%<HiLim>
  LimOffsRange4 : NxtrLim/LimStat_f32  LoLim=PINIONAGLOWLIM_HWDEG_F32  HiLim=PINIONAGHILIM_HWDEG_F32
      settings: AttributesFormatString=|
      | Low Limit: %<LoLim>
      | High Limit:%<HiLim>
  LimOffsRange5 : NxtrLim/LimStat_f32  LoLim=PINIONAGLOWLIM_HWDEG_F32  HiLim=PINIONAGHILIM_HWDEG_F32
      settings: AttributesFormatString=|
      | Low Limit: %<LoLim>
      | High Limit:%<HiLim>
  LimOffsRange7 : NxtrLim/LimStat_f32  LoLim=PINIONVELLOWLIM_HWRADPERSEC_F32  HiLim=PINIONVELHILIM_HWRADPERSEC_F32
      settings: AttributesFormatString=|
      | Low Limit: %<LoLim>
      | High Limit:%<HiLim>
  LimOffsRange8 : NxtrLim/LimStat_f32  LoLim=HWVELLOWLIM_HWRADPERSEC_F32  HiLim=HWVELHILIM_HWRADPERSEC_F32
      settings: AttributesFormatString=|
      | Low Limit: %<LoLim>
      | High Limit:%<HiLim>
  LimOffsRange9 : NxtrLim/LimStat_f32  LoLim=PINIONAGCONFLOWLIM_ULS_F32  HiLim=PINIONAGCONFHILIM_ULS_F32
      settings: AttributesFormatString=|
      | Low Limit: %<LoLim>
      | High Limit:%<HiLim>
  HwAgFinal : Outport
  PinionAg : Outport  Port=2
  PinionAgConf : Outport  Port=3
  HwAgNotCorrd : Outport  Port=4
  HwAgToSerlCom : Outport  Port=5
  HwAgVldToSerlCom : Outport  Port=6
  PinionVel : Outport  Port=7
  HwVel : Outport  Port=8
  PinionVelConf : Outport  Port=9
  HwVelToSerlCom : Outport  Port=10
  wires:
  LimOffsRange3/1 -> PinionAgConf/1
  Add/1 -> LimOffsRange2/1
  LimOffsRange1/1 -> FltInj_f32 client/1(Sig)
  Constant/1 -> FltInj_f32 client/2("LocnKey  ")
  LimOffsRange5/1 -> FltInj_f32 client1/1(Sig)
  FltInj_f32 client1/1(Sig_Out) -> HwAgToSerlCom/1
  Constant1/1 -> FltInj_f32 client1/2("LocnKey  ")
  FltInj_f32 client/1(Sig_Out) -> Add/1, PinionAg/1
  LimOffsRange4/1 -> HwAgNotCorrd/1
  HwAgSnsrlsConf/1 -> HwAgArbn/4(HwAgSnsrlsConf)
  HwAgIdptSig/1 -> HwAgArbn/2(HwAgIdptSig)
  CmplncErrPinionToHw/1 -> Add/2
  LimOffsRange2/1 -> HwAgFinal/1
  HwAgSnsrls/1 -> HwAgArbn/3(HwAgSnsrls)
  HwAg/1 -> HwAgArbn/5(HwAg)
  HwAgArbn/1(PinionAg) -> LimOffsRange1/1
  HwAgArbn/2(PinionAgConf) -> LimOffsRange3/1
  HwAgArbn/4(HwAgToSerlCom) -> LimOffsRange5/1
  HwAgArbn/3(HwAgNotCorrd) -> LimOffsRange4/1
  HwAgCorrd/1 -> HwAgArbn/1(HwAgCorrd)
  MotVelCrf/1 -> HwAgArbn/6(MotVelCrf)
  MotVelVld/1 -> HwAgArbn/7(MotVelVld)
  HwTq/1 -> HwAgArbn/8(HwTq)
  HwAgArbn/6(PinionVel) -> LimOffsRange7/1
  HwAgArbn/7(HwVel) -> LimOffsRange8/1
  HwAgArbn/8(PinionVelConf) -> LimOffsRange9/1
  HwAgArbn/9(HwVelToSerlCom) -> LimOffsRange10/1
  HwAgArbn/5(HwAgVldToSerlCom) -> HwAgVldToSerlCom/1
  LimOffsRange7/1 -> PinionVel/1
  LimOffsRange8/1 -> HwVel/1
  LimOffsRange9/1 -> PinionVelConf/1
  LimOffsRange10/1 -> HwVelToSerlCom/1

== system SF045A_HwAgSysArbn/HwAgSysArbnInit1/CopyRight2 ==

== system SF045A_HwAgSysArbn/HwAgSysArbnPer1/CopyRight2 ==

== system SF045A_HwAgSysArbn/HwAgSysArbn/HwAgSysArbnInit1/CopyRight2 ==

== system SF045A_HwAgSysArbn/HwAgSysArbn/HwAgSysArbnInit1/GetRefTmr100MicroSec32bit ==
  note: 1 count = 100 uSec
  note: seconds
  note: microseconds
  note: counts
  note: Wrap-to-zero
  note: GetRefTmr100MicroSec32bit
  CopyRight2 : Subsystem  Description=|  mask(Copyright Information){none=on}
      | Copyright info block.                                               
      |                                                                     
      | Place copyright information at the top of every subsystem in design.
      mask prompts: none "No parameters"
      mask help: Place copyright information at the top of every subsystem in design.
      mask Display:
      | NxtrConf = 'Nexteer Confidential';
      | 
      | sys = bdroot; %handle for the current model ("system")
      | first = get_param(sys,'Created');
      | if(isempty(first))
      |     first = datestr(now,'yyyy');
      | else
      |     first = first(end-3:end);  %year is last four digits
      | end
      | 
      | last = get_param(sys,'LastModifiedDate');
      | if isempty(last)
      |     last = datestr(now,'yyyy');
      | else
      |     last = last(end-3:end);
      | end
      | 
      | if strcmp(first,last)
      |     fprintf('%s -- Copyright %s Nexteer',NxtrConf,first)
      | else
      |     fprintf('%s -- %s%s- %s Nexteer',NxtrConf,char(169),first,last)
      | end
  Count per uSec : Constant  Value=0.01
  Data Store Read1 : DataStoreRead  DataStoreName=SimnTi
  Data Type Conversion1 : DataTypeConversion  OutDataTypeStr=uint32
  Divide1 : Product  Inputs=**
  Divide2 : Product  Inputs=*/
  Max Counts : Constant  Value=2^32-1
  Product1 : Product
  Product2 : Product
  Rounding : Rounding
  Subtract1 : Sum  Inputs=+-
  uSec per Sec : Constant  Value=1000000
  RefTmr : Outport
  wires:
  Product2/1 -> Subtract1/2
  Subtract1/1 -> Data Type Conversion1/1
  Rounding/1 -> Product2/1
  Divide2/1 -> Rounding/1
  Max Counts/1 -> Divide2/2, Product2/2
  Divide1/1 -> Divide2/1, Subtract1/1
  Product1/1 -> Divide1/1
  Data Store Read1/1 -> Product1/1
  Count per uSec/1 -> Divide1/2
  uSec per Sec/1 -> Product1/2
  Data Type Conversion1/1 -> RefTmr/1

== system SF045A_HwAgSysArbn/HwAgSysArbn/HwAgSysArbnInit1/Kinematic Integrity ==
  NtcNr : Inport
  NtcStInfo : Inport  Port=2
  NtcSts : Inport  Port=3
  DebStep : Inport  Port=4
  SetNtcSts : Subsystem  RequirementInfo={} %GIDa_16f23167_f05b_46c3_9fcc_0dcafd7bcf3c  TreatAsAtomicUnit=on
      settings: RTWSystemCode=Inline
  wires:
  NtcStInfo/1 -> SetNtcSts/2(NtcStInfo)
  DebStep/1 -> SetNtcSts/4(DebStep)
  NtcSts/1 -> SetNtcSts/3(NtcSts)
  NtcNr/1 -> SetNtcSts/1(NtcNr)  "NtcNr"

== system SF045A_HwAgSysArbn/HwAgSysArbn/HwAgSysArbnPer1/CopyRight2 ==

== system SF045A_HwAgSysArbn/HwAgSysArbn/HwAgSysArbnPer1/FltInj_f32 client ==
  note: FltInj_f32
  note: 1) Only subsystems can be added as variant choices at this level
      | 2) Blocks cannot be connected at this level as connectivity is
      | automatically determined at simulation, based on the active variant
  note: Created Aug 18, 2015
      | Kevin Derry
  Sig : Inport  OutDataTypeStr=single
  "LocnKey  " : Inport  Port=2  OutDataTypeStr=uint16
  CodeGen : Subsystem  VariantControl=FLTINJENA == STD_ON
  CopyRight1 : Subsystem  Description=|  mask(Copyright Information){none=on}
      | Copyright info block.                                               
      |                                                                     
      | Place copyright information at the top of every subsystem in design.
      mask prompts: none "No parameters"
      mask help: Place copyright information at the top of every subsystem in design.
      mask Display:
      | NxtrConf = 'Nexteer Confidential';
      | 
      | sys = bdroot; %handle for the current model ("system")
      | first = get_param(sys,'Created');
      | if(isempty(first))
      |     first = datestr(now,'yyyy');
      | else
      |     first = first(end-3:end);  %year is last four digits
      | end
      | 
      | last = get_param(sys,'LastModifiedDate');
      | if isempty(last)
      |     last = datestr(now,'yyyy');
      | else
      |     last = last(end-3:end);
      | end
      | 
      | if strcmp(first,last)
      |     fprintf('%s -- Copyright %s Nexteer',NxtrConf,first)
      | else
      |     fprintf('%s -- %s%s- %s Nexteer',NxtrConf,char(169),first,last)
      | end
  CopyRight2 : Subsystem  Description=|  mask(Copyright Information){none=on}
      | Copyright info block.                                               
      |                                                                     
      | Place copyright information at the top of every subsystem in design.
      mask prompts: none "No parameters"
      mask help: Place copyright information at the top of every subsystem in design.
      mask Display:
      | NxtrConf = 'Nexteer Confidential';
      | 
      | sys = bdroot; %handle for the current model ("system")
      | first = get_param(sys,'Created');
      | if(isempty(first))
      |     first = datestr(now,'yyyy');
      | else
      |     first = first(end-3:end);  %year is last four digits
      | end
      | 
      | last = get_param(sys,'LastModifiedDate');
      | if isempty(last)
      |     last = datestr(now,'yyyy');
      | else
      |     last = last(end-3:end);
      | end
      | 
      | if strcmp(first,last)
      |     fprintf('%s -- Copyright %s Nexteer',NxtrConf,first)
      | else
      |     fprintf('%s -- %s%s- %s Nexteer',NxtrConf,char(169),first,last)
      | end
  Sim : Subsystem  TreatAsAtomicUnit=on  VariantControl=FLTINJENA ~= STD_ON  mask(Fault_Injection){}
      mask help: Simulation mode is just a pass-thru.
  Sig_Out : Outport  OutDataTypeStr=single

== system SF045A_HwAgSysArbn/HwAgSysArbn/HwAgSysArbnPer1/FltInj_f32 client1 ==
  note: Created Aug 18, 2015
      | Kevin Derry
  note: 1) Only subsystems can be added as variant choices at this level
      | 2) Blocks cannot be connected at this level as connectivity is
      | automatically determined at simulation, based on the active variant
  note: FltInj_f32
  Sig : Inport  OutDataTypeStr=single
  "LocnKey  " : Inport  Port=2  OutDataTypeStr=uint16
  CodeGen : Subsystem  VariantControl=FLTINJENA == STD_ON
  CopyRight1 : Subsystem  Description=|  mask(Copyright Information){none=on}
      | Copyright info block.                                               
      |                                                                     
      | Place copyright information at the top of every subsystem in design.
      mask prompts: none "No parameters"
      mask help: Place copyright information at the top of every subsystem in design.
      mask Display:
      | NxtrConf = 'Nexteer Confidential';
      | 
      | sys = bdroot; %handle for the current model ("system")
      | first = get_param(sys,'Created');
      | if(isempty(first))
      |     first = datestr(now,'yyyy');
      | else
      |     first = first(end-3:end);  %year is last four digits
      | end
      | 
      | last = get_param(sys,'LastModifiedDate');
      | if isempty(last)
      |     last = datestr(now,'yyyy');
      | else
      |     last = last(end-3:end);
      | end
      | 
      | if strcmp(first,last)
      |     fprintf('%s -- Copyright %s Nexteer',NxtrConf,first)
      | else
      |     fprintf('%s -- %s%s- %s Nexteer',NxtrConf,char(169),first,last)
      | end
  CopyRight2 : Subsystem  Description=|  mask(Copyright Information){none=on}
      | Copyright info block.                                               
      |                                                                     
      | Place copyright information at the top of every subsystem in design.
      mask prompts: none "No parameters"
      mask help: Place copyright information at the top of every subsystem in design.
      mask Display:
      | NxtrConf = 'Nexteer Confidential';
      | 
      | sys = bdroot; %handle for the current model ("system")
      | first = get_param(sys,'Created');
      | if(isempty(first))
      |     first = datestr(now,'yyyy');
      | else
      |     first = first(end-3:end);  %year is last four digits
      | end
      | 
      | last = get_param(sys,'LastModifiedDate');
      | if isempty(last)
      |     last = datestr(now,'yyyy');
      | else
      |     last = last(end-3:end);
      | end
      | 
      | if strcmp(first,last)
      |     fprintf('%s -- Copyright %s Nexteer',NxtrConf,first)
      | else
      |     fprintf('%s -- %s%s- %s Nexteer',NxtrConf,char(169),first,last)
      | end
  Sim : Subsystem  TreatAsAtomicUnit=on  VariantControl=FLTINJENA ~= STD_ON  mask(Fault_Injection){}
      mask help: Simulation mode is just a pass-thru.
  Sig_Out : Outport  OutDataTypeStr=single
